simulink model "Adjustable_Power_Supply_Block_Diagram"  (R2025a)
settings: Solver=VariableStepAuto  StartTime=0.0  StopTime=10.0  RelTol=1e-3
settings Model: Creator=Jabro  LastModifiedBy=Jabro

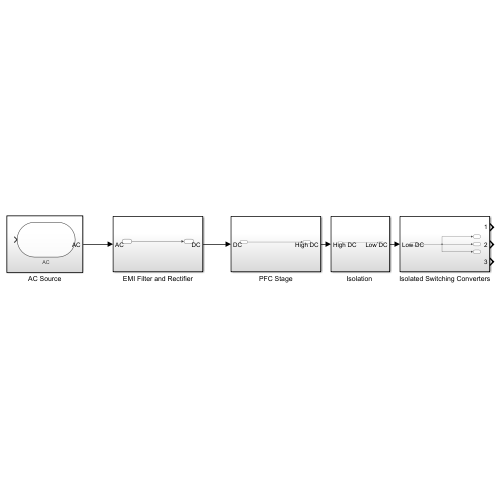
[thumbnail: Simulink's stored preview of the top-level diagram]
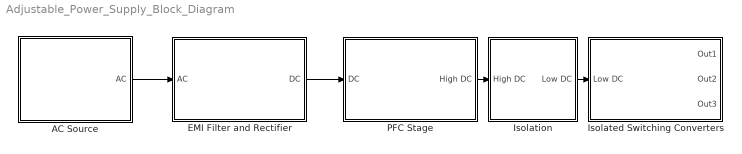
== system Adjustable_Power_Supply_Block_Diagram ==
  AC Source : Subsystem
  EMI Filter and Rectifier : Subsystem
  Isolated Switching Converters : Subsystem
  "Isolation " : Subsystem
  PFC Stage : Subsystem
  wires:
  AC Source/1(AC) -> EMI Filter and Rectifier/1(AC)
  EMI Filter and Rectifier/1(DC) -> PFC Stage/1(DC)
  PFC Stage/1(High DC) -> "Isolation "/1(High DC)
  "Isolation "/1(Low DC) -> Isolated Switching Converters/1(Low DC)

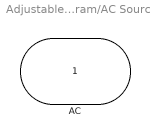
== system Adjustable_Power_Supply_Block_Diagram/AC Source ==
  AC : Outport

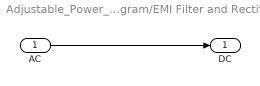
== system Adjustable_Power_Supply_Block_Diagram/EMI Filter and Rectifier ==
  AC : Inport
  DC : Outport
  wires:
  AC/1 -> DC/1

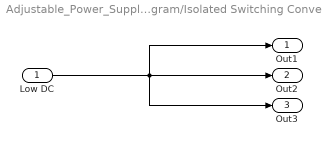
== system Adjustable_Power_Supply_Block_Diagram/Isolated Switching Converters ==
  Low DC : Inport
  Out1 : Outport
  Out2 : Outport  Port=2
  Out3 : Outport  Port=3
  wires:
  Low DC/1 -> Out3/1, Out1/1, Out2/1

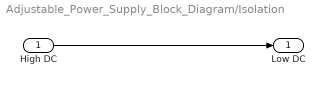
== system Adjustable_Power_Supply_Block_Diagram/Isolation  ==
  High DC : Inport
  Low DC : Outport
  wires:
  High DC/1 -> Low DC/1

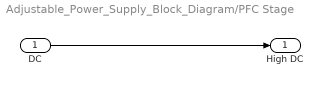
== system Adjustable_Power_Supply_Block_Diagram/PFC Stage ==
  DC : Inport
  High DC : Outport
  wires:
  DC/1 -> High DC/1
